simulink model "comms_test_cap_subsys"  (Simulink 7.5)
settings: Solver=ode45  StartTime=0.0  StopTime=10*30  FixedStep=.0001  MaxStep=.02  RelTol=1e-3
InitFcn:
  | Ts=0.02;
settings Model: Creator=jporter  LastModifiedBy=Joe P
settings OptimizationCC: InitFltsAndDblsToZero=on
settings DebuggingCC: StrictBusMsg=Warning

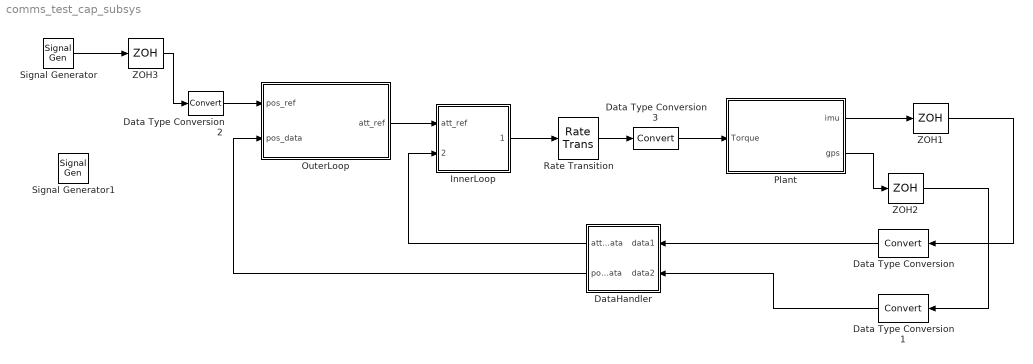
== system comms_test_cap_subsys ==
  Data Type Conversion{,1..3} (4 alike) : DataTypeConversion  OutDataType=sfix(16)  OutScaling=2^0
  DataHandler : Subsystem
  InnerLoop : Subsystem
  OuterLoop : Subsystem
  Plant : Subsystem
  Rate Transition : RateTransition
  Signal Generator : SignalGenerator  WaveForm=square  Amplitude=ones(1,4)  Frequency=1/100000
  Signal Generator1 : SignalGenerator  Amplitude=ones(1,4)  Frequency=1/30
  ZOH1 : ZeroOrderHold  SampleTime=Ts
  ZOH2 : ZeroOrderHold  SampleTime=Ts
  ZOH3 : ZeroOrderHold  SampleTime=Ts
  wires:
  InnerLoop/1(Torque) -> Rate Transition/1
  Data Type Conversion3/1 -> Plant/1(Torque)
  Rate Transition/1 -> Data Type Conversion3/1
  ZOH1/1 -> Data Type Conversion/1
  Plant/1(imu) -> ZOH1/1
  OuterLoop/1(att_ref) -> InnerLoop/1(att_ref)
  ZOH2/1 -> Data Type Conversion1/1
  Plant/2(gps) -> ZOH2/1
  Data Type Conversion/1 -> DataHandler/1(data1)
  Data Type Conversion1/1 -> DataHandler/2(data2)
  DataHandler/1(att_data) -> InnerLoop/2(att_data)
  Signal Generator/1 -> ZOH3/1
  Data Type Conversion2/1 -> OuterLoop/1(pos_ref)
  ZOH3/1 -> Data Type Conversion2/1
  DataHandler/2(pos_data) -> OuterLoop/2(pos_data)

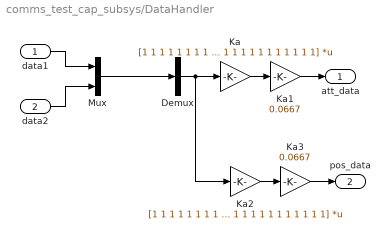
== system comms_test_cap_subsys/DataHandler ==
  data1 : Inport  PortDimensions=9  DataType=single  OutDataTypeStr=single
  data2 : Inport  Port=2  PortDimensions=6  DataType=single  OutDataTypeStr=single
  Demux : Demux  Outputs=1
  Ka : Gain  Gain=[1 1 1 1 1 1 1 1 1 1 1 1 1 1 1; 1 1 1 1 1 1 1 1 1 1 1 1 1 1 1; 1 1 1 1 1 1 1 1 1 1 1 1 1 1 1; 1 1 1 1 1 1 1 1 1 1 1 1 1 1 1; 1 1 1 1 1 1 1 1 1 1 1 1 1 1 1; 1 1 1 1 1 1 1 1 1 1 1 1 1 1 1]  Multiplication=Matrix(K*u)  ParameterDataTypeMode=single  ParameterDataType=sfix(16)  ParameterScaling=2^0  ParamDataTypeStr=single  OutDataType=sfix(16)  OutScaling=2^0
  Ka1 : Gain  Gain=0.0667  ParameterDataTypeMode=single  ParameterDataType=sfix(16)  ParameterScaling=2^0  ParamDataTypeStr=single  OutDataType=sfix(16)  OutScaling=2^0
  Ka2 : Gain  Gain=[1 1 1 1 1 1 1 1 1 1 1 1 1 1 1; 1 1 1 1 1 1 1 1 1 1 1 1 1 1 1; 1 1 1 1 1 1 1 1 1 1 1 1 1 1 1; 1 1 1 1 1 1 1 1 1 1 1 1 1 1 1; 1 1 1 1 1 1 1 1 1 1 1 1 1 1 1; 1 1 1 1 1 1 1 1 1 1 1 1 1 1 1; 1 1 1 1 1 1 1 1 1 1 1 1 1 1 1; 1 1 1 1 1 1 1 1 1 1 1 1 1 1 1; 1 1 1 1 1 1 1 1 1 1 1 1 1 1 1; 1 1 1 1 1 1 1 1 1 1 1 1 1 1 1; 1 1 1 1 1 1 1 1 1 1 1 1 1 1 1; 1 1 1 1 1 1 1 1 1 1 1 1 1 1 1]  Multiplication=Matrix(K*u)  ParameterDataTypeMode=single  ParameterDataType=sfix(16)  ParameterScaling=2^0  ParamDataTypeStr=single  OutDataType=sfix(16)  OutScaling=2^0
  Ka3 : Gain  Gain=0.0667  ParameterDataTypeMode=single  ParameterDataType=sfix(16)  ParameterScaling=2^0  ParamDataTypeStr=single  OutDataType=sfix(16)  OutScaling=2^0
  Mux : Mux  Inputs=2
  att_data : Outport  DataType=single  OutDataTypeStr=single
  pos_data : Outport  Port=2  DataType=single  OutDataTypeStr=single
  wires:
  Ka/1 -> Ka1/1
  data1/1 -> Mux/1
  data2/1 -> Mux/2
  Mux/1 -> Demux/1
  Ka1/1 -> att_data/1
  Demux/1 -> Ka/1, Ka2/1
  Ka2/1 -> Ka3/1
  Ka3/1 -> pos_data/1

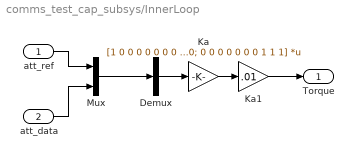
== system comms_test_cap_subsys/InnerLoop ==
  att_ref : Inport  PortDimensions=4  DataType=single  OutDataTypeStr=single
  att_data : Inport  Port=2  PortDimensions=6  DataType=single  OutDataTypeStr=single
  Demux : Demux  Outputs=1
  Ka : Gain  Gain=[1 0 0 0 0 0 0 0 0 0; 0 1 1 1 0 0 0 0 0 0; 0 0 0 0 1 1 1 0 0 0; 0 0 0 0 0 0 0 1 1 1]  Multiplication=Matrix(K*u)  ParameterDataTypeMode=single  ParameterDataType=sfix(16)  ParameterScaling=2^0  ParamDataTypeStr=single  OutDataType=sfix(16)  OutScaling=2^0
  Ka1 : Gain  Gain=.01  ParameterDataTypeMode=single  ParameterDataType=sfix(16)  ParameterScaling=2^0  ParamDataTypeStr=single  OutDataType=sfix(16)  OutScaling=2^0
  Mux : Mux  Inputs=2
  Torque : Outport  DataType=single  OutDataTypeStr=single
  wires:
  Ka/1 -> Ka1/1
  att_ref/1 -> Mux/1
  att_data/1 -> Mux/2
  Mux/1 -> Demux/1
  Ka1/1 -> Torque/1
  Demux/1 -> Ka/1

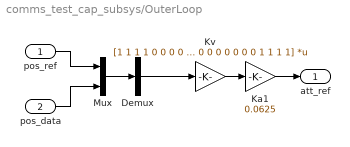
== system comms_test_cap_subsys/OuterLoop ==
  pos_ref : Inport  PortDimensions=4  DataType=single  OutDataTypeStr=single
  pos_data : Inport  Port=2  PortDimensions=12  DataType=single  OutDataTypeStr=single
  Demux : Demux  Outputs=1
  Ka1 : Gain  Gain=0.0625  ParameterDataTypeMode=single  ParameterDataType=sfix(16)  ParameterScaling=2^0  ParamDataTypeStr=single  OutDataType=sfix(16)  OutScaling=2^0
  Kv : Gain  Gain=[1 1 1 1 0 0 0 0 0 0 0 0 0 0 0 0; 0 0 0 0 1 1 1 1 0 0 0 0 0 0 0 0; 0 0 0 0 0 0 0 0 1 1 1 1 0 0 0 0; 0 0 0 0 0 0 0 0 0 0 0 0 1 1 1 1]  Multiplication=Matrix(K*u)  ParameterDataTypeMode=single  ParameterDataType=sfix(16)  ParameterScaling=2^0  ParamDataTypeStr=single  OutDataType=sfix(16)  OutScaling=2^0
  Mux : Mux  Inputs=2
  att_ref : Outport  DataType=single  OutDataTypeStr=single
  wires:
  Kv/1 -> Ka1/1
  pos_ref/1 -> Mux/1
  pos_data/1 -> Mux/2
  Ka1/1 -> att_ref/1
  Mux/1 -> Demux/1
  Demux/1 -> Kv/1

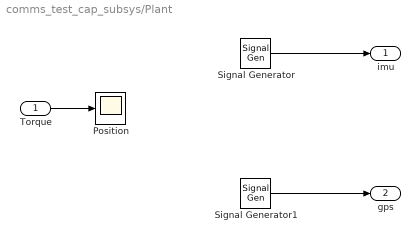
== system comms_test_cap_subsys/Plant ==
  Torque : Inport
  Position : Scope
      settings: YMin=-20  YMax=20  SaveName=ScopeData7
  Signal Generator : SignalGenerator  Amplitude=ones(1,9)  Frequency=1/30
  Signal Generator1 : SignalGenerator  Amplitude=ones(1,6)  Frequency=1/30
  imu : Outport
  gps : Outport  Port=2
  wires:
  Signal Generator/1 -> imu/1
  Torque/1 -> Position/1
  Signal Generator1/1 -> gps/1
